simulink model "Turbine_model_2017a"  (R2020a)
settings: Solver=VariableStepAuto  StartTime=0.0  StopTime=5  RelTol=1e-3
values from neighbouring files (symbols this model uses):
  R = 36.8000    (= 36.8)    [Untitled2.m]
undefined symbols (not defined in the file or in its folder): G, magnitude, T
libraries: simulink x1
settings Model: Creator=ander  LastModifiedBy=delfi
settings DebuggingCC: SFMachineParentedDataDiag=error  ArithmeticOperatorsInVariantConditions=warning
settings SFSimCC: CustomCodeUndefinedFunction=UseInterfaceOnly
settings CodeAppCC: StateflowObjectComments=on

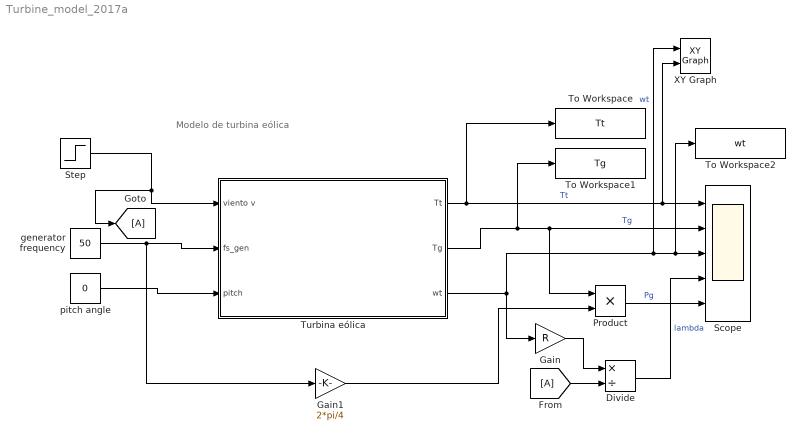
== system Turbine_model_2017a ==
  note: Modelo de turbina eólica
  Divide : Product  Inputs=*/
  Gain : Gain  Gain=R
  Gain1 : Gain  Gain=2*pi/4
  Product : Product
  Scope : Scope  NumInputPorts=5
  Step : Step  Before=5  After=5  SampleTime=0
  To Workspace : ToWorkspace  VariableName=Tt  SampleTime=-1
      settings: Save2DSignal=2-D array (concatenate along first dimension)
  To Workspace1 : ToWorkspace  VariableName=Tg  SampleTime=-1
      settings: Save2DSignal=2-D array (concatenate along first dimension)
  To Workspace2 : ToWorkspace  VariableName=wt  SampleTime=-1
      settings: Save2DSignal=2-D array (concatenate along first dimension)
  Turbina eólica : Subsystem
  XY Graph : simulink/Sinks/XY Graph  xmin=0  xmax=3  ymin=0  ymax=15e5  st=-1
  generator frequency : Constant  Value=50
  pitch angle : Constant  Value=0
  wires:
  Turbina eólica/1(Tt) -> To Workspace/1, XY Graph/2, Scope/1  "Tt"
  Turbina eólica/2(Tg) -> To Workspace1/1, Product/1, Scope/2  "Tg"
  Turbina eólica/3(wt) -> XY Graph/1, To Workspace2/1, Scope/3, Gain/1  "wt"
  generator frequency/1 -> Gain1/1, Turbina eólica/2(fs_gen)
  pitch angle/1 -> Turbina eólica/3(pitch)
  Step/1 -> [A], Turbina eólica/1(viento v)
  Gain/1 -> Divide/1
  [A] -> Divide/2
  Divide/1 -> Scope/4  "lambda"
  Product/1 -> Scope/5  "Pg"
  Gain1/1 -> Product/2

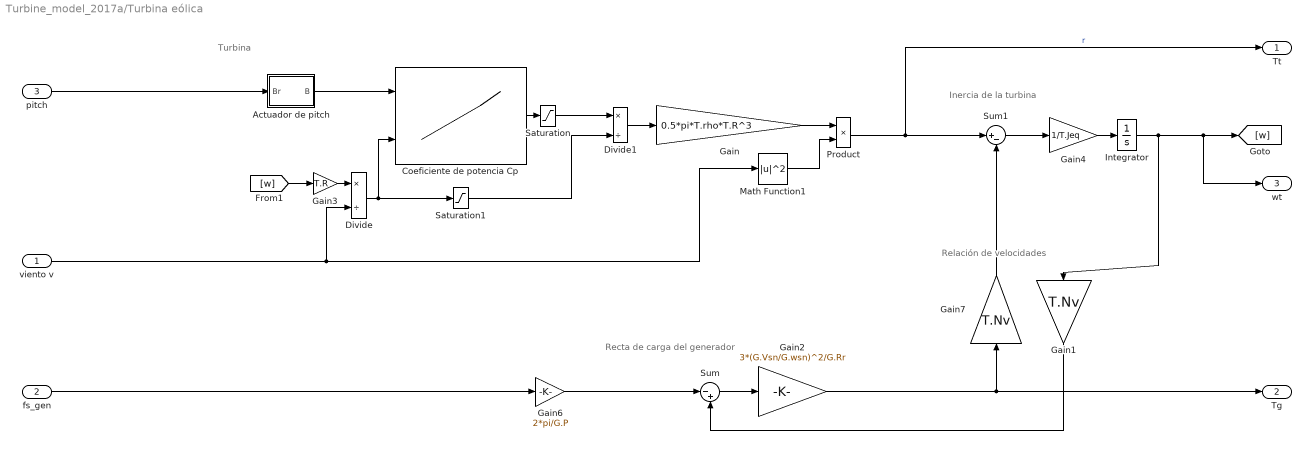
== system Turbine_model_2017a/Turbina eólica ==
  note: Relación de velocidades
  note: Turbina
  note: Inercia de la turbina
  note: Recta de carga del generador
  viento v : Inport
  fs_gen : Inport  Port=2
  pitch : Inport  Port=3
  Actuador de pitch : Subsystem
  Coeficiente de potencia Cp : Lookup_n-D  BreakpointsForDimension1=T.pitch  BreakpointsForDimension2=T.tsr  Table=T.Cp  InterpMethod=Cubic spline  InternalRulePriority=Speed  OutMin=[0]  OutMax=[0.5]  RndMeth=Simplest  SaturateOnIntegerOverflow=on  InputSameDT=on
  Divide : Product  Inputs=*/
  Divide1 : Product  Inputs=*/
  Gain : Gain  Gain=0.5*pi*T.rho*T.R^3
  Gain1 : Gain  Gain=T.Nv
  Gain2 : Gain  Gain=3*(G.Vsn/G.wsn)^2/G.Rr
  Gain3 : Gain  Gain=T.R
  Gain4 : Gain  Gain=1/T.Jeq
  Gain6 : Gain  Gain=2*pi/G.P
  Gain7 : Gain  Gain=T.Nv
  Integrator : Integrator  InitialCondition=G.wsn/T.Nv
  Math Function1 : Math  Operator=magnitude^2  SignedPower=on  SaturateOnIntegerOverflow=on
  Product : Product
  Saturation : Saturate  LowerLimit=0
  Saturation1 : Saturate  UpperLimit=inf  LowerLimit=0.1
  Sum : Sum  Inputs=|-+
  Sum1 : Sum  Inputs=|+-
  Tt : Outport
  Tg : Outport  Port=2
  wt : Outport  Port=3
  wires:
  Coeficiente de potencia Cp/1 -> Saturation/1
  fs_gen/1 -> Gain6/1
  Divide/1 -> Coeficiente de potencia Cp/2, Saturation1/1
  Integrator/1 -> Gain1/1, wt/1, [w]
  Gain3/1 -> Divide/1
  viento v/1 -> Divide/2, Math Function1/1
  Product/1 -> Tt/1, Sum1/1  "r"
  Gain2/1 -> Tg/1, Gain7/1
  Sum1/1 -> Gain4/1
  Gain7/1 -> Sum1/2
  [w] -> Gain3/1
  Math Function1/1 -> Product/2
  Saturation1/1 -> Divide1/2
  Saturation/1 -> Divide1/1
  Gain1/1 -> Sum/2
  Sum/1 -> Gain2/1
  Divide1/1 -> Gain/1
  Gain/1 -> Product/1
  Gain4/1 -> Integrator/1
  Gain6/1 -> Sum/1
  pitch/1 -> Actuador de pitch/1(Br)
  Actuador de pitch/1(B) -> Coeficiente de potencia Cp/1

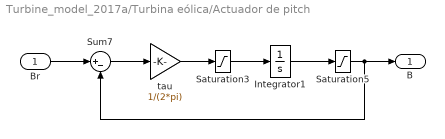
== system Turbine_model_2017a/Turbina eólica/Actuador de pitch ==
  Br : Inport
  Integrator1 : Integrator
  Saturation3 : Saturate  UpperLimit=10  LowerLimit=-10
  Saturation5 : Saturate  UpperLimit=30  LowerLimit=0
  Sum7 : Sum  Inputs=|+-
  tau : Gain  Gain=1/(2*pi)
  B : Outport
  wires:
  Saturation5/1 -> B/1, Sum7/2
  Integrator1/1 -> Saturation5/1
  tau/1 -> Saturation3/1
  Saturation3/1 -> Integrator1/1
  Sum7/1 -> tau/1
  Br/1 -> Sum7/1
